simulink model "hscc_AbstractFuelControl_M3_Stateflow"  (R2014a)
settings: Solver=ode15s  StartTime=0.0  StopTime=10  RelTol=1e-3
settings Model: Creator=cfan10  LastModifiedBy=Luan Nguyen
settings DataIOCC: LimitDataPoints=off  SaveFormat=StructureWithTime  SaveOutput=off  SaveTime=off
settings DebuggingCC: UnderspecifiedInitializationDetection=Classic

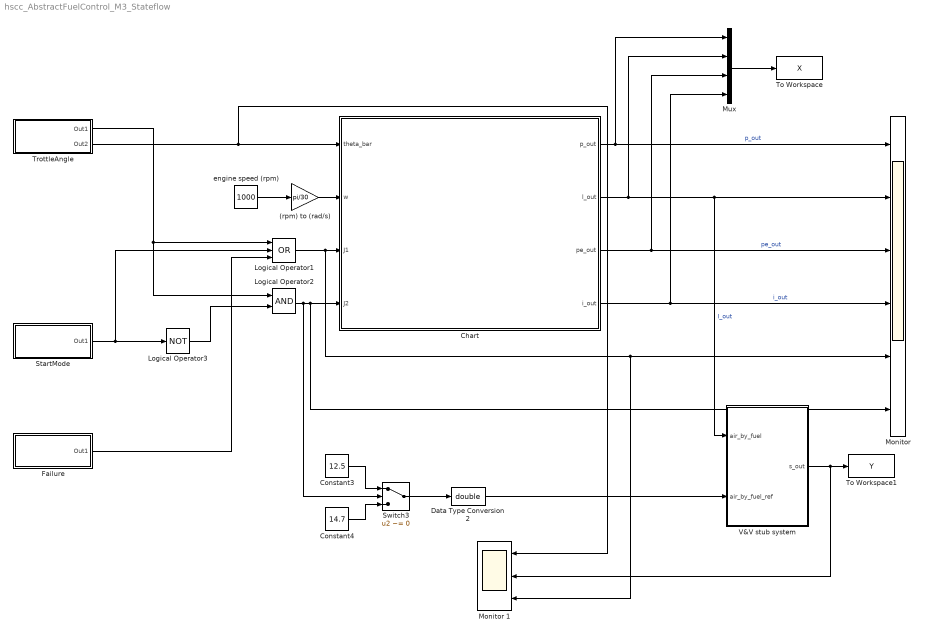
== system hscc_AbstractFuelControl_M3_Stateflow ==
  (rpm) to (rad/s) : Gain  Gain=pi/30
  Chart : Stateflow chart  TreatAsAtomicUnit=on
  Constant3 : Constant  Value=12.5
  Constant4 : Constant  Value=14.7
  Data Type Conversion2 : DataTypeConversion  OutDataTypeStr=double
  Failure : Subsystem  TreatAsAtomicUnit=on
  Logical Operator1 : Logic  Operator=OR  Inputs=3  AllPortsSameDT=off  OutDataTypeStr=boolean
  Logical Operator2 : Logic  AllPortsSameDT=off  OutDataTypeStr=boolean
  Logical Operator3 : Logic  Operator=NOT  Inputs=3  AllPortsSameDT=off  OutDataTypeStr=boolean
  "Monitor " : Scope  NumInputPorts=6
      settings: TimeRange=50  YMin=1.04864~14.685~0.867643~0.0127~-1~-1  YMax=1.04864~14.695~0.867643~0.0136~1~1  SaveName=ScopeData2
  Monitor 1 : Scope  NumInputPorts=3
      settings: TimeRange=50  YMin=0~-0.01~0  YMax=55~0.01~1
  Mux : Mux
  StartMode : Subsystem  TreatAsAtomicUnit=on
  Switch3 : Switch  Criteria=u2 ~= 0
  To Workspace : ToWorkspace  VariableName=X  SaveFormat=Timeseries  SampleTime=-1
  To Workspace1 : ToWorkspace  VariableName=Y  SaveFormat=Timeseries  SampleTime=-1
  TrottleAngle : Subsystem  Description=Trottle angle  TreatAsAtomicUnit=on
  V&V stub system : Subsystem  TreatAsAtomicUnit=on
  engine speed (rpm) : Constant  Description=[1000, 3000]  Value=1000
      settings: AttributesFormatString=%<Description>
  wires:
  engine speed (rpm)/1 -> (rpm) to (rad/s)/1
  (rpm) to (rad/s)/1 -> Chart/2(w)
  TrottleAngle/2(Out2) -> Monitor 1/1, Chart/1(theta_bar)
  TrottleAngle/1(Out1) -> Logical Operator2/1, Logical Operator1/1
  StartMode/1(Out1) -> Logical Operator1/2, Logical Operator3/1
  Failure/1(Out1) -> Logical Operator1/3
  Logical Operator1/1 -> Monitor 1/3, "Monitor "/5, Chart/3(J1)
  Logical Operator3/1 -> Logical Operator2/2
  Chart/2(l_out) -> Mux/2, V&V stub system/1("air_by_fuel "), "Monitor "/2  "I_out"
  Chart/3(pe_out) -> Mux/3, "Monitor "/3  "pe_out"
  Chart/4(i_out) -> Mux/4, "Monitor "/4  "i_out"
  Mux/1 -> To Workspace/1
  Chart/1(p_out) -> Mux/1, "Monitor "/1  "p_out"
  Switch3/1 -> Data Type Conversion2/1
  Constant3/1 -> Switch3/1
  Constant4/1 -> Switch3/3
  Logical Operator2/1 -> Switch3/2, "Monitor "/6, Chart/4(J2)
  Data Type Conversion2/1 -> V&V stub system/2(air_by_fuel_ref)
  V&V stub system/1("s_out ") -> Monitor 1/2, To Workspace1/1

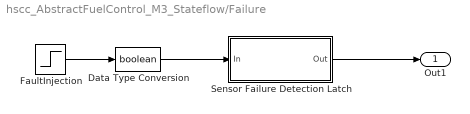
== system hscc_AbstractFuelControl_M3_Stateflow/Failure ==
  Data Type Conversion : DataTypeConversion  OutDataTypeStr=boolean
  FaultInjection : Step  Time=60  SampleTime=0
      settings: AttributesFormatString=1: Failure\n0: Normal
  Sensor Failure Detection Latch : Subsystem  TreatAsAtomicUnit=on
  Out1 : Outport
  wires:
  Data Type Conversion/1 -> Sensor Failure Detection Latch/1(In)
  FaultInjection/1 -> Data Type Conversion/1
  Sensor Failure Detection Latch/1(Out) -> Out1/1

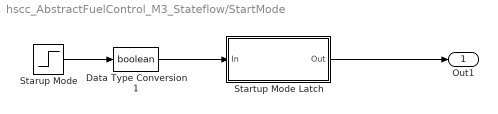
== system hscc_AbstractFuelControl_M3_Stateflow/StartMode ==
  Data Type Conversion1 : DataTypeConversion  OutDataTypeStr=boolean
  Startup Mode Latch : Subsystem  TreatAsAtomicUnit=on
  Starup Mode : Step  Time=10  Before=1  After=0  SampleTime=0
  Out1 : Outport
  wires:
  Data Type Conversion1/1 -> Startup Mode Latch/1(In)
  Starup Mode/1 -> Data Type Conversion1/1
  Startup Mode Latch/1(Out) -> Out1/1

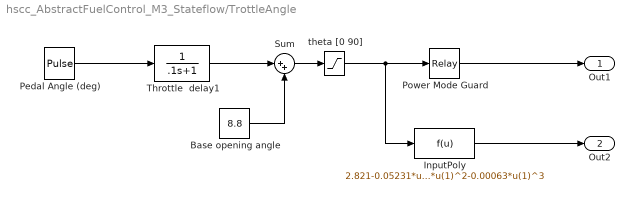
== system hscc_AbstractFuelControl_M3_Stateflow/TrottleAngle ==
  Base opening angle : Constant  Value=8.8
  InputPoly : Fcn  Expr=2.821-0.05231*u(1)+0.10299*u(1)^2-0.00063*u(1)^3
  Pedal Angle (deg) : DiscretePulseGenerator  PulseType=Time based  Amplitude=53.468  Period=20.5223  PulseWidth=50  PhaseDelay=3
  Power Mode Guard : Relay  OnSwitchValue=70  OffSwitchValue=50  SampleTime=0.01
  Sum : Sum  Inputs=|++
  Throttle  delay1 : TransferFcn  Denominator=[.1 1]
  theta [0 90] : Saturate  UpperLimit=90  LowerLimit=0
  Out1 : Outport
  Out2 : Outport  Port=2
  wires:
  Base opening angle/1 -> Sum/2
  Pedal Angle (deg)/1 -> Throttle  delay1/1
  Throttle  delay1/1 -> Sum/1
  Sum/1 -> theta [0 90]/1
  theta [0 90]/1 -> InputPoly/1, Power Mode Guard/1
  Power Mode Guard/1 -> Out1/1
  InputPoly/1 -> Out2/1

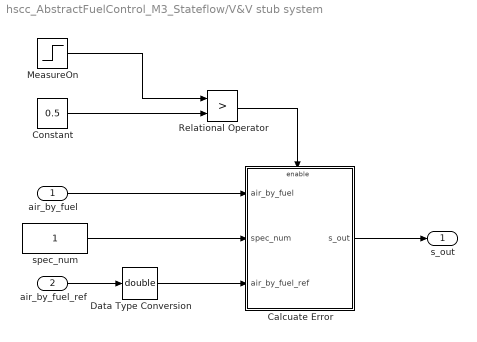
== system hscc_AbstractFuelControl_M3_Stateflow/V&V stub system ==
  "air_by_fuel " : Inport  OutDataTypeStr=double
  air_by_fuel_ref : Inport  Port=2
  Calcuate Error : Subsystem  Priority=20  TreatAsAtomicUnit=on
  Constant : Constant  Value=0.5
  Data Type Conversion : DataTypeConversion  OutDataTypeStr=double
  MeasureOn : Step  SampleTime=0
  Relational Operator : RelationalOperator  Operator=>  OutDataTypeStr=boolean
  spec_num : Constant  OutDataTypeStr=uint8
  "s_out " : Outport
  wires:
  Calcuate Error/1("s_out ") -> "s_out "/1
  MeasureOn/1 -> Relational Operator/1
  Constant/1 -> Relational Operator/2
  Relational Operator/1 -> Calcuate Error/Enable
  spec_num/1 -> Calcuate Error/2(spec_num)
  "air_by_fuel "/1 -> Calcuate Error/1("air_by_fuel ")
  air_by_fuel_ref/1 -> Data Type Conversion/1
  Data Type Conversion/1 -> Calcuate Error/3(air_by_fuel_ref)

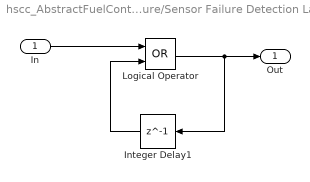
== system hscc_AbstractFuelControl_M3_Stateflow/Failure/Sensor Failure Detection Latch ==
  In : Inport
  Integer Delay1 : Delay  DelayLength=1  SampleTime=0.01
  Logical Operator : Logic  Operator=OR  AllPortsSameDT=off
  Out : Outport
  wires:
  Logical Operator/1 -> Out/1, Integer Delay1/1
  Integer Delay1/1 -> Logical Operator/2
  In/1 -> Logical Operator/1

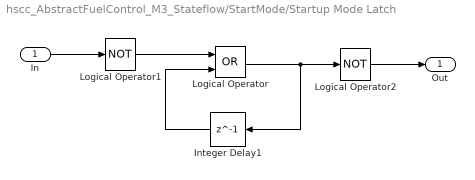
== system hscc_AbstractFuelControl_M3_Stateflow/StartMode/Startup Mode Latch ==
  In : Inport
  Integer Delay1 : Delay  DelayLength=1  SampleTime=0.01
  Logical Operator : Logic  Operator=OR  AllPortsSameDT=off
  Logical Operator1 : Logic  Operator=NOT  AllPortsSameDT=off
  Logical Operator2 : Logic  Operator=NOT  AllPortsSameDT=off
  Out : Outport
  wires:
  In/1 -> Logical Operator1/1
  Integer Delay1/1 -> Logical Operator/2
  Logical Operator/1 -> Integer Delay1/1, Logical Operator2/1
  Logical Operator1/1 -> Logical Operator/1
  Logical Operator2/1 -> Out/1

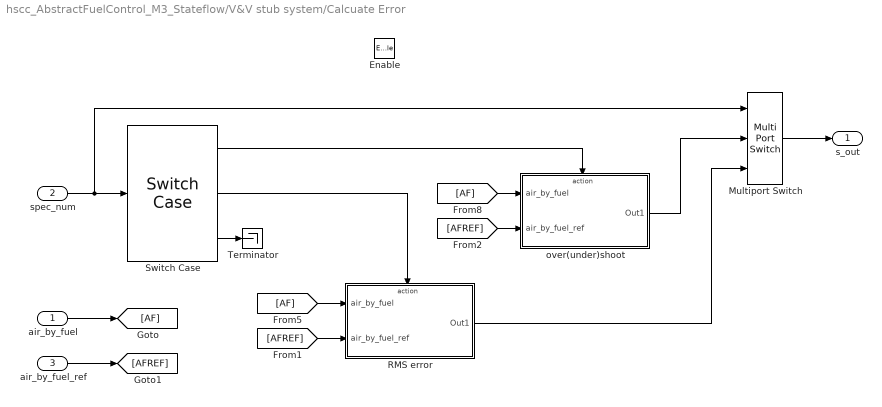
== system hscc_AbstractFuelControl_M3_Stateflow/V&V stub system/Calcuate Error ==
  "air_by_fuel " : Inport
  spec_num : Inport  Port=2  OutDataTypeStr=uint8
  air_by_fuel_ref : Inport  Port=3
  Enable : EnablePort
  Multiport Switch : MultiPortSwitch  Inputs=2
  RMS error : Subsystem  TreatAsAtomicUnit=on
  Switch Case : SwitchCase  CaseConditions={1,2}
  Terminator : Terminator
  over(under)shoot : Subsystem  TreatAsAtomicUnit=on
  "s_out " : Outport
  wires:
  "air_by_fuel "/1 -> [AF]
  spec_num/1 -> Multiport Switch/1, Switch Case/1
  Switch Case/1 -> over(under)shoot/Action
  [AF] -> over(under)shoot/1("air_by_fuel ")
  Switch Case/2 -> RMS error/Action
  [AF] -> RMS error/1("air_by_fuel ")
  Multiport Switch/1 -> "s_out "/1
  over(under)shoot/1(Out1) -> Multiport Switch/2
  RMS error/1(Out1) -> Multiport Switch/3
  Switch Case/3 -> Terminator/1
  air_by_fuel_ref/1 -> [AFREF]
  [AFREF] -> over(under)shoot/2(air_by_fuel_ref)
  [AFREF] -> RMS error/2(air_by_fuel_ref)

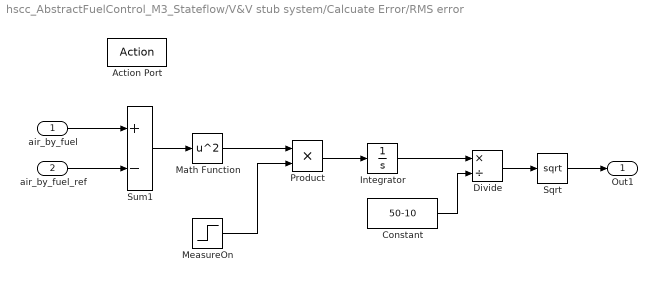
== system hscc_AbstractFuelControl_M3_Stateflow/V&V stub system/Calcuate Error/RMS error ==
  "air_by_fuel " : Inport
  air_by_fuel_ref : Inport  Port=2
  Action Port : ActionPort  ActionType=case
  Constant : Constant  Value=50-10
  Divide : Product  Inputs=*/
  Integrator : Integrator
  Math Function : Math  Operator=square  SaturateOnIntegerOverflow=on
  MeasureOn : Step  Time=10  SampleTime=0
  Product : Product
  Sqrt : Sqrt  SaturateOnIntegerOverflow=on
  Sum1 : Sum  Inputs=+-  OutDataTypeStr=Inherit: Inherit via back propagation  RndMeth=Simplest  InputSameDT=on
  Out1 : Outport
  wires:
  Sum1/1 -> Math Function/1
  Math Function/1 -> Product/1
  "air_by_fuel "/1 -> Sum1/1
  Constant/1 -> Divide/2
  air_by_fuel_ref/1 -> Sum1/2
  MeasureOn/1 -> Product/2
  Product/1 -> Integrator/1
  Divide/1 -> Sqrt/1
  Sqrt/1 -> Out1/1
  Integrator/1 -> Divide/1

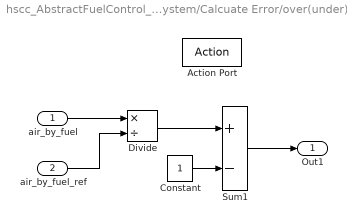
== system hscc_AbstractFuelControl_M3_Stateflow/V&V stub system/Calcuate Error/over(under)shoot ==
  "air_by_fuel " : Inport
  air_by_fuel_ref : Inport  Port=2
  Action Port : ActionPort  ActionType=case
  Constant : Constant
  Divide : Product  Inputs=*/
  Sum1 : Sum  Inputs=+-  OutDataTypeStr=Inherit: Inherit via back propagation  RndMeth=Simplest  InputSameDT=on
  Out1 : Outport
  wires:
  "air_by_fuel "/1 -> Divide/1
  Divide/1 -> Sum1/1
  Constant/1 -> Sum1/2
  Sum1/1 -> Out1/1
  air_by_fuel_ref/1 -> Divide/2

== stateflow chart hscc_AbstractFuelControl_M3_Stateflow/Chart ==
  settings: updateMethod=CONTINUOUS
  state start
    entry:
    p = 0.6353;
    l = 14.7;
    pe = 0.5573;
    i = 0.017;
  state main_dynamic01
    during:
    p_dot = c1*(2*theta_bar*(c20*p*p+c21*p+c22)-c12*(c2+c3*w*p+c4*w*p*p+c5*w*w*p));
    l_dot = 4*(c15+c16*c25*((1/12.5)*(c2+c3*w*pe+c4*w*pe*pe+c5*pe*w*w))+c17*c25*c25*((1/12.5)*(c2+c3*w*pe+c4*w*pe*pe+c5*pe*w*w))*((1/12.5)*(c2+c3*w*pe+c4*w*pe*pe+c5*pe*w*w))+c18*(c12*(c2+c3*w*p+c4*w*p*p+c5*p*w*w)) +c19*(c12*(c2+c3*w*p+c4*w*p*p+c5*p*w*w)) *c25*((1/12.5)*(c2+c3*w*pe+c4*w*pe*pe+c5*pe*w*w))-l);
    pe_dot = c1*(2*c23*(theta_bar)*(c20*p*p+c21*p+c22)-(c2+c3*w*pe+c4*w*pe*pe+c5*pe*w*w));
    i_dot = c14*(c24*l-c11);
    p_out = p;
    l_out = l;
    pe_out = pe;
    i_out = i;
  state main_dynamic00
    during:
    p_dot = c1*(2*theta_bar*(c20*p*p+c21*p+c22)-c12*(c2+c3*w*p+c4*w*p*p+c5*w*w*p));
    l_dot = 4*(c15+c16*c25*((1/c11)*(1+i+c13*(c24*l-c11))*(c2+c3*w*pe+c4*w*pe*pe+c5*pe*w*w))+c17*c25*c25*((1/c11)*(1+i+c13*(c24*l-c11))*(c2+c3*w*pe+c4*w*pe*pe+c5*pe*w*w))*((1/c11)*(1+i+c13*(c24*l-c11))*(c2+c3*w*pe+c4*w*pe*pe+c5*pe*w*w))+c18*(c12*(c2+c3*w*p+c4*w*p*p+c5*p*w*w)) +c19*(c12*(c2+c3*w*p+c4*w*p*p+c5*p*w*w)) *c25*((1/c11)*(1+i+c13*(c24*l-c11))*(c2+c3*w*pe+c4*w*pe*pe+c5*pe*w*w))-l);
    pe_dot = c1*(2*c23*(theta_bar)*(c20*p*p+c21*p+c22)-(c2+c3*w*pe+c4*w*pe*pe+c5*pe*w*w));
    i_dot = c14*(c24*l-c11);
    p_out = p;
    l_out = l;
    pe_out = pe;
    i_out = i;
  state main_dynamic11
    during:
    p_dot = c1*(2*theta_bar*(c20*p*p+c21*p+c22)-c12*(c2+c3*w*p+c4*w*p*p+c5*w*w*p));
    l_dot = 4*(c15+c16*c25*((1/12.5)*(c2+c3*w*pe+c4*w*pe*pe+c5*pe*w*w))+c17*c25*c25*((1/12.5)*(c2+c3*w*pe+c4*w*pe*pe+c5*pe*w*w))*((1/12.5)*(c2+c3*w*pe+c4*w*pe*pe+c5*pe*w*w))+c18*(c12*(c2+c3*w*p+c4*w*p*p+c5*p*w*w)) +c19*(c12*(c2+c3*w*p+c4*w*p*p+c5*p*w*w)) *c25*((1/12.5)*(c2+c3*w*pe+c4*w*pe*pe+c5*pe*w*w))-l);
    pe_dot = c1*(2*c23*(theta_bar)*(c20*p*p+c21*p+c22)-(c2+c3*w*pe+c4*w*pe*pe+c5*pe*w*w));
    i_dot = 0;
    p_out = p;
    l_out = l;
    pe_out = pe;
    i_out = i;
  state main_dynamic10
    during:
    p_dot = c1*(2*theta_bar*(c20*p*p+c21*p+c22)-c12*(c2+c3*w*p+c4*w*p*p+c5*w*w*p));
    l_dot = 4*(c15+c16*c25*((1/c11)*(c2+c3*w*pe+c4*w*pe*pe+c5*pe*w*w))+c17*c25*c25*((1/c11)*(c2+c3*w*pe+c4*w*pe*pe+c5*pe*w*w))*((1/c11)*(c2+c3*w*pe+c4*w*pe*pe+c5*pe*w*w))+c18*(c12*(c2+c3*w*p+c4*w*p*p+c5*p*w*w)) +c19*(c12*(c2+c3*w*p+c4*w*p*p+c5*p*w*w)) *c25*((1/c11)*(c2+c3*w*pe+c4*w*pe*pe+c5*pe*w*w))-l);
    pe_dot = c1*(2*c23*(theta_bar)*(c20*p*p+c21*p+c22)-(c2+c3*w*pe+c4*w*pe*pe+c5*pe*w*w));
    i_dot = 0;
    p_out = p;
    l_out = l;
    pe_out = pe;
    i_out = i;
  (default) -> start : {l = 14.7;}
  start -> main_dynamic10 [order 3] : [J1==1&&J2==0]
  start -> main_dynamic00 [order 1] : [J1==0&&J2==0]
  start -> main_dynamic11 [order 4] : [J1==1&&J2==1]
  start -> main_dynamic01 [order 2] : [J1==0&&J2==1]
  main_dynamic01 -> main_dynamic00 [order 2] : [J1==0&&J2==0]
  main_dynamic00 -> main_dynamic01 [order 2] : [J1==0&&J2==1]
  main_dynamic01 -> main_dynamic10 [order 1] : [J1==1&&J2==0]
  main_dynamic10 -> main_dynamic01 [order 2] : [J1==0&&J2==1]
  main_dynamic11 -> main_dynamic01 [order 3] : [J1==0&&J2==1]
  main_dynamic01 -> main_dynamic11 [order 3] : [J1==1&&J2==1]
  main_dynamic10 -> main_dynamic00 [order 1] : [J1==0&&J2==0]
  main_dynamic00 -> main_dynamic10 [order 1] : [J1==1&&J2==0]
  main_dynamic11 -> main_dynamic00 [order 2] : [J1==0&&J2==0]
  main_dynamic00 -> main_dynamic11 [order 3] : [J1==1&&J2==1]
  main_dynamic11 -> main_dynamic10 [order 1] : [J1==1&&J2==0]
  main_dynamic10 -> main_dynamic11 [order 3] : [J1==1&&J2==1]
  data: p local double =0.6353; l local double =14.7; pe local double =0.5573; i local double =0.017; p_out output double; l_out output double; pe_out output double; i_out output double; theta_bar input double; w input double; J1 input boolean; J2 input boolean
  data p settings: updateMethod=SF_CONTINUOUS_TIME_DATA
  data l settings: updateMethod=SF_CONTINUOUS_TIME_DATA
  data pe settings: updateMethod=SF_CONTINUOUS_TIME_DATA
  data i settings: updateMethod=SF_CONTINUOUS_TIME_DATA
